simulink model "MPC_control"  (R2025a)
settings: Solver=VariableStepAuto  StartTime=0.0  StopTime=7000  RelTol=1e-3
undefined symbols (not defined in the file): A1, B1, C1, D1, SIG_FINAL_VALUE, SIG_INIT_VALUE, STEP_TIME
libraries: mpclib x1
settings Model: Creator=Mick  LastModifiedBy=Mick

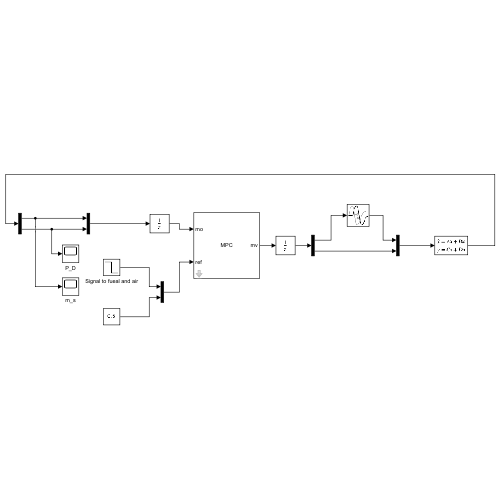
[thumbnail: Simulink's stored preview of the top-level diagram]
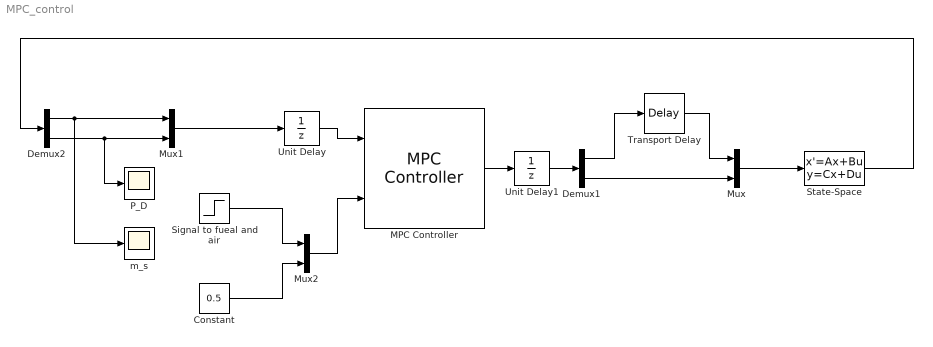
== system MPC_control ==
  Constant : Constant  Value=0.5
  Demux1 : Demux  Outputs=2
  Demux2 : Demux  Outputs=2
  MPC Controller : mpclib/MPC Controller  SCDEnableBlockLinearizationSpecification=on  mpcobj=mpcobj  is_multiple=0  enable_value=0  return_u0=off  updateMPCinCallerWorkspace=on  md_inport=off  mv_inport=off  uref_inport=off  return_cost=off  return_mvseq=off  return_qpstatus=off  return_xseq=off  return_state=off  return_ovseq=off  state_inport=off  umin_inport=off  umax_inport=off  ymin_inport=off  ymax_inport=off  cc_inport=off  ywt_inport=off  uwt_inport=off  duwt_inport=off  rhoeps_inport=off  pm_inport=off  MaximumP=10  HorizonChoice=FixedHorizon  n_ts=1  n_p=10  n_mv=2  n_md=0  n_ud=0  n_mo=2  n_uo=0  BlockDataType=double  SampleTimeInherited=off  switch_inport=off
  Mux : Mux  Inputs=2
  Mux1 : Mux  Inputs=2
  Mux2 : Mux  Inputs=2
  P_D : Scope
      settings: ActiveDisplayYMinimum=-0.081754091306359952  ActiveDisplayYMaximum=0.73578682175723964
  Signal to fueal and air : Step  Time=STEP_TIME  Before=SIG_INIT_VALUE  After=SIG_FINAL_VALUE  SampleTime=0
  State-Space : StateSpace  A=A1  B=B1  C=C1  D=D1  InitialCondition=0
  Transport Delay : TransportDelay
  Unit Delay : UnitDelay  SampleTime=-1  HasFrameUpgradeWarning=on
  Unit Delay1 : UnitDelay  SampleTime=-1  HasFrameUpgradeWarning=on
  m_s : Scope
      settings: ActiveDisplayYMinimum=-0.15798918260309783  ActiveDisplayYMaximum=1.4219026434278808
  wires:
  Mux/1 -> State-Space/1
  Transport Delay/1 -> Mux/1
  Unit Delay1/1 -> Demux1/1
  Demux1/1 -> Transport Delay/1
  Demux1/2 -> Mux/2
  Demux2/1 -> m_s/1, Mux1/1
  Demux2/2 -> P_D/1, Mux1/2
  Mux1/1 -> Unit Delay/1
  Signal to fueal and air/1 -> Mux2/1
  Constant/1 -> Mux2/2
  State-Space/1 -> Demux2/1
  MPC Controller/1 -> Unit Delay1/1
  Mux2/1 -> MPC Controller/2
  Unit Delay/1 -> MPC Controller/1
